simulink model "Buck_Boost_Converter"  (Simulink 7.5)
settings: Solver=ode45  StartTime=0.0  StopTime=0.3  RelTol=1e-3
libraries: powerlib x11, simulink x1
settings Model: Creator=Quang Thien  LastModifiedBy=Quang Thien

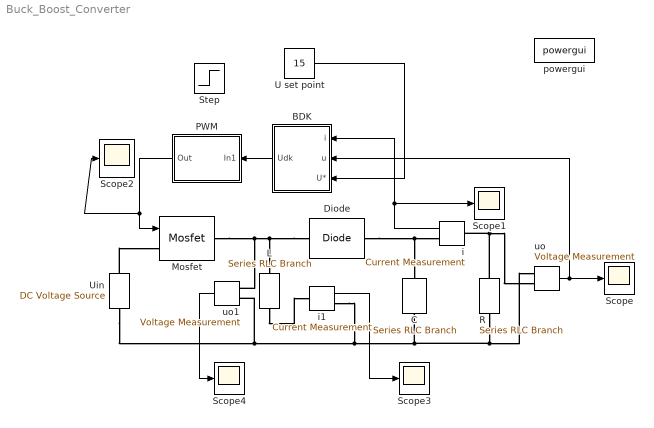
== system Buck_Boost_Converter ==
  BDK : Subsystem
  C : powerlib/Elements/Series RLC Branch  DialogController=POWERSYS.PowerSysDialog  PhysicalDomain=powersysdomain  SubClassName=unknown  LeftPortType=p1  RightPortType=p1  LConnTagsString=__new0  RConnTagsString=__new0  BranchType=RC  Resistance=0.01  Inductance=1e-3  SetiL0=off  InitialCurrent=0  Capacitance=697e-6  Setx0=off  InitialVoltage=0  Measurements=None
  Diode : powerlib/Power Electronics/Diode  DialogController=POWERSYS.PowerSysDialog  SystemSampleTime=-1  Ron=1e-6  Lon=0  Vf=0  IC=0  UseSnubber=off  Rs=500  Cs=250e-9  Measurements=off
  L : powerlib/Elements/Series RLC Branch  DialogController=POWERSYS.PowerSysDialog  PhysicalDomain=powersysdomain  SubClassName=unknown  LeftPortType=p1  RightPortType=p1  LConnTagsString=__new0  RConnTagsString=__new0  BranchType=L  Resistance=1  Inductance=100e-6  SetiL0=off  InitialCurrent=0  Capacitance=1e-6  Setx0=off  InitialVoltage=0  Measurements=None
  Mosfet : powerlib/Power Electronics/Mosfet  DialogController=POWERSYS.PowerSysDialog  SystemSampleTime=-1  Ron=1e-6  Lon=0  Rd=1e-6  Vfd=0  IC=0  Rs=1e5  Cs=inf  Measurements=off
  PWM : Subsystem
  R : powerlib/Elements/Series RLC Branch  DialogController=POWERSYS.PowerSysDialog  PhysicalDomain=powersysdomain  SubClassName=unknown  LeftPortType=p1  RightPortType=p1  LConnTagsString=__new0  RConnTagsString=__new0  BranchType=R  Resistance=2.25  Inductance=1e-3  SetiL0=off  InitialCurrent=0  Capacitance=1e-6  Setx0=off  InitialVoltage=0  Measurements=None
  Scope{,1..4} (5 alike) : Scope
      Scope settings: YMin=13.4935  YMax=13.501  MaxDataPoints=500000  SampleInput=on  SampleTime=50e-6
      Scope1 settings: YMin=13.4935  YMax=13.501  SaveName=ScopeData3  MaxDataPoints=500000  SampleInput=on  SampleTime=50e-6
      Scope2 settings: TimeRange=0.00012  YMin=0  YMax=1
      Scope3 settings: YMin=13.4935  YMax=13.501  SaveName=ScopeData5  MaxDataPoints=500000  SampleInput=on  SampleTime=50e-6
      Scope4 settings: YMin=13.4935  YMax=13.501  SaveName=ScopeData6  MaxDataPoints=500000  SampleInput=on  SampleTime=50e-6
  Step : Step  Time=0.05  Before=0.385  After=0.385  SampleTime=0
  U set point : Constant  Value=15  OutDataType=fixdt(1, 16)  OutScaling=2^0
  Uin : powerlib/Electrical Sources/DC Voltage Source  DialogController=POWERSYS.PowerSysDialog  SystemSampleTime=-1  Amplitude=24  Measurements=None
  i : powerlib/Measurements/Current Measurement  DialogController=POWERSYS.PowerSysDialog  SystemSampleTime=-1  PhasorSimulation=off  OutputType=Complex  PSBequivalent=0
  i1 : powerlib/Measurements/Current Measurement  DialogController=POWERSYS.PowerSysDialog  SystemSampleTime=-1  PhasorSimulation=off  OutputType=Complex  PSBequivalent=0
  powergui : powerlib/powergui  SystemSampleTime=-1  SimulationMode=Continuous  SampleTime=200e-6  frequency=60  SPID=on  DisableSnubberDevices=off  DisableRonSwitches=off  DisableVfSwitches=off  SwTol=0  Interpol=off  frequencyindice=0  echomessages=off  HookPort=off  DisplayEquations=off  FunctionMessages=off  EnableUseOfTLC=off  x0status=blocks  RestoreLinks=warning  ResistiveCurrentMeasurement=off  Frange=[0:2:500]  Ylog=off  Xlog=on  ShowGrid=off  save=off  variable=ZData  structure=psbconverter_str1  ZoomFFT=off  StartTime=0.05  cycles=3  DisplayStyle=2  fundamental=50  FreqAxis=on  MaxFrequency=1000  frequencyindicesteady=1  RmsSteady=1  display=off  Ts=0  methode=off
  uo : powerlib/Measurements/Voltage Measurement  DialogController=POWERSYS.PowerSysDialog  SystemSampleTime=-1  PhasorSimulation=off  OutputType=Complex  PSBequivalent=0
  uo1 : powerlib/Measurements/Voltage Measurement  DialogController=POWERSYS.PowerSysDialog  SystemSampleTime=-1  PhasorSimulation=off  OutputType=Complex  PSBequivalent=0
  wires:
  uo/1 -> Scope/1, BDK/2(u)
  PWM/1(Out) -> Scope2/1, Mosfet/1
  i1/1 -> Scope3/1
  i/1 -> BDK/1(i), Scope1/1
  U set point/1 -> BDK/3(U*)
  uo1/1 -> Scope4/1
  BDK/1(Udk) -> PWM/1(In1)
  connections:
  Uin/LConn1 -- i1/RConn1 -- C/RConn1 -- R/RConn1 -- uo/LConn1 -- uo1/LConn2
  Diode/RConn1 -- L/LConn1 -- uo1/LConn1 -- Mosfet/RConn1
  R/LConn1 -- uo/LConn2 -- i/LConn1
  Uin/RConn1 -- Mosfet/LConn1
  L/RConn1 -- i1/LConn1
  Diode/LConn1 -- i/RConn1 -- C/LConn1

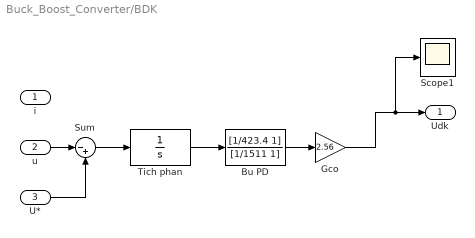
== system Buck_Boost_Converter/BDK ==
  i : Inport  OutDataType=fixdt(1, 16)  OutScaling=2^0
  u : Inport  Port=2  OutDataType=fixdt(1, 16)  OutScaling=2^0
  U* : Inport  Port=3  OutDataType=fixdt(1, 16)  OutScaling=2^0
  Bu PD : TransferFcn  Numerator=[1/423.4 1]  Denominator=[1/1511 1]
  Gco : Gain  Gain=2.56  ParameterDataType=fixdt(1, 16)  ParameterScaling=2^0  OutDataType=fixdt(1, 16)  OutScaling=2^0
  Scope1 : Scope
      settings: TimeRange=0.00012  YMin=0  YMax=1
  Sum : Sum  Inputs=|-+  OutDataType=fixdt(1, 16)  OutScaling=2^0
  Tich phan : TransferFcn  Denominator=[1 0]
  Udk : Outport  OutDataType=fixdt(1, 16)  OutScaling=2^0
  wires:
  u/1 -> Sum/1
  U*/1 -> Sum/2
  Gco/1 -> Udk/1, Scope1/1
  Bu PD/1 -> Gco/1
  Sum/1 -> Tich phan/1
  Tich phan/1 -> Bu PD/1

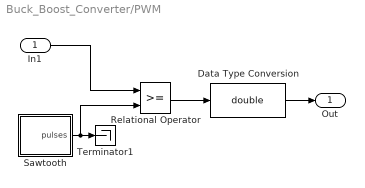
== system Buck_Boost_Converter/PWM ==
  In1 : Inport
  Data Type Conversion : DataTypeConversion  OutDataTypeMode=double  OutDataTypeStr=double
  Relational Operator : RelationalOperator  LogicOutDataTypeMode=boolean  OutDataTypeStr=boolean
  Sawtooth : Subsystem
  Terminator1 : Terminator
  Out : Outport
  wires:
  Sawtooth/1(pulses) -> Relational Operator/2, Terminator1/1
  Data Type Conversion/1 -> Out/1
  Relational Operator/1 -> Data Type Conversion/1
  In1/1 -> Relational Operator/1

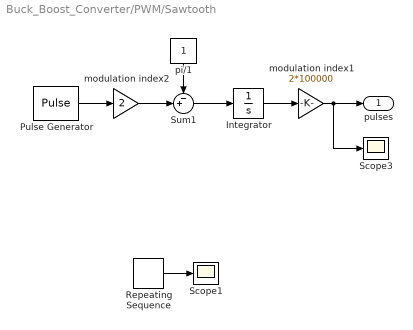
== system Buck_Boost_Converter/PWM/Sawtooth ==
  Integrator : Integrator
  Pulse Generator : DiscretePulseGenerator  PulseType=Time based  Amplitude=1  Period=1/100000  PulseWidth=50  PhaseDelay=0  SampleTime=1
  Repeating Sequence : simulink/Sources/Repeating Sequence  SystemSampleTime=-1  rep_seq_t=[0 1e-5]  rep_seq_y=[0 1]
  Scope1 : Scope
      settings: TimeRange=4.5  YMin=-0.25  YMax=4.25  SaveName=ScopeData2
  Scope3 : Scope
      settings: TimeRange=4.5  YMin=-0.25  YMax=4.25  SaveName=ScopeData4
  Sum1 : Sum  Inputs=-+|  SaturateOnIntegerOverflow=on  InputSameDT=on  OutDataTypeStr=Inherit: Same as first input
  modulation index1 : Gain  Gain=2*100000  SaturateOnIntegerOverflow=on  OutDataTypeStr=Inherit: Same as input  ParamDataTypeStr=Inherit: Same as input
  modulation index2 : Gain  Gain=2  SaturateOnIntegerOverflow=on  OutDataTypeStr=Inherit: Same as input  ParamDataTypeStr=Inherit: Same as input
  pi/1 : Constant
  pulses : Outport
  wires:
  Repeating Sequence/1 -> Scope1/1
  pi/1/1 -> Sum1/1
  modulation index2/1 -> Sum1/2
  Sum1/1 -> Integrator/1
  modulation index1/1 -> Scope3/1, pulses/1
  Integrator/1 -> modulation index1/1
  Pulse Generator/1 -> modulation index2/1
